simulink model "pulse_generator"  (R2021a)
(part 3 of 11)

  out_3_stop_6 : Subsystem  Tag=xps:sw_reg  AncestorBlock=xps_library/Memory/software_register  mask(swreg){io_dir=From Processor, io_delay=0, init_val=0, sample_period=1, names=reg, bitwidths=32, bin_pts=0, arith_types=0, sim_port=on, show_format=on}
      mask prompts: io_dir "I/O direction"; io_delay "I/O delay"; init_val "Initial Value"; sample_period "Sample period"; names "Bitfield names [msb...lsb]"; bitwidths "Bitfield widths"; bin_pts "Bitfield binary pts"; arith_types "Bitfield types, ufix=0, fix=1, bool=2"; sim_port "Provide sim input/output?"; show_format "Print format string?"
      mask help: A 32-bit software-accessible register. Can be divided into bitfields of varying widths and types using the fields in the block mask.
      mask init:
      | swreg_init(gcb)
      settings: AttributesFormatString=1input:uf32.0 = 32 bits
      mask TypeOptions io_dir: To Processor | From Processor
      mask Callback io_dir:
      | mask_enables = get_param(gcb, 'MaskEnables');
      | mask_names = get_param(gcb, 'MaskNames');
      | if strcmp(get_param(gcb, 'io_dir'), 'To Processor'),
      |     mask_enables{ismember(mask_names, 'sample_period')} = 'off';
      | else
      |     mask_enables{ismember(mask_names, 'sample_period')} = 'on';
      | end
      | set_param(gcb, 'MaskEnables', mask_enables);
      mask DialogControl ParameterTabVar0 Prompt: Setup
  out_3_stop_7 : Subsystem  Tag=xps:sw_reg  AncestorBlock=xps_library/Memory/software_register  mask(swreg){io_dir=From Processor, io_delay=0, init_val=0, sample_period=1, names=reg, bitwidths=32, bin_pts=0, arith_types=0, sim_port=on, show_format=on}
      mask prompts: io_dir "I/O direction"; io_delay "I/O delay"; init_val "Initial Value"; sample_period "Sample period"; names "Bitfield names [msb...lsb]"; bitwidths "Bitfield widths"; bin_pts "Bitfield binary pts"; arith_types "Bitfield types, ufix=0, fix=1, bool=2"; sim_port "Provide sim input/output?"; show_format "Print format string?"
      mask help: A 32-bit software-accessible register. Can be divided into bitfields of varying widths and types using the fields in the block mask.
      mask init:
      | swreg_init(gcb)
      settings: AttributesFormatString=1input:uf32.0 = 32 bits
      mask TypeOptions io_dir: To Processor | From Processor
      mask Callback io_dir:
      | mask_enables = get_param(gcb, 'MaskEnables');
      | mask_names = get_param(gcb, 'MaskNames');
      | if strcmp(get_param(gcb, 'io_dir'), 'To Processor'),
      |     mask_enables{ismember(mask_names, 'sample_period')} = 'off';
      | else
      |     mask_enables{ismember(mask_names, 'sample_period')} = 'on';
      | end
      | set_param(gcb, 'MaskEnables', mask_enables);
      mask DialogControl ParameterTabVar0 Prompt: Setup
  out_3_stop_8 : Subsystem  Tag=xps:sw_reg  AncestorBlock=xps_library/Memory/software_register  mask(swreg){io_dir=From Processor, io_delay=0, init_val=0, sample_period=1, names=reg, bitwidths=32, bin_pts=0, arith_types=0, sim_port=on, show_format=on}
      mask prompts: io_dir "I/O direction"; io_delay "I/O delay"; init_val "Initial Value"; sample_period "Sample period"; names "Bitfield names [msb...lsb]"; bitwidths "Bitfield widths"; bin_pts "Bitfield binary pts"; arith_types "Bitfield types, ufix=0, fix=1, bool=2"; sim_port "Provide sim input/output?"; show_format "Print format string?"
      mask help: A 32-bit software-accessible register. Can be divided into bitfields of varying widths and types using the fields in the block mask.
      mask init:
      | swreg_init(gcb)
      settings: AttributesFormatString=1input:uf32.0 = 32 bits
      mask TypeOptions io_dir: To Processor | From Processor
      mask Callback io_dir:
      | mask_enables = get_param(gcb, 'MaskEnables');
      | mask_names = get_param(gcb, 'MaskNames');
      | if strcmp(get_param(gcb, 'io_dir'), 'To Processor'),
      |     mask_enables{ismember(mask_names, 'sample_period')} = 'off';
      | else
      |     mask_enables{ismember(mask_names, 'sample_period')} = 'on';
      | end
      | set_param(gcb, 'MaskEnables', mask_enables);
      mask DialogControl ParameterTabVar0 Prompt: Setup
  out_3_stop_9 : Subsystem  Tag=xps:sw_reg  AncestorBlock=xps_library/Memory/software_register  mask(swreg){io_dir=From Processor, io_delay=0, init_val=0, sample_period=1, names=reg, bitwidths=32, bin_pts=0, arith_types=0, sim_port=on, show_format=on}
      mask prompts: io_dir "I/O direction"; io_delay "I/O delay"; init_val "Initial Value"; sample_period "Sample period"; names "Bitfield names [msb...lsb]"; bitwidths "Bitfield widths"; bin_pts "Bitfield binary pts"; arith_types "Bitfield types, ufix=0, fix=1, bool=2"; sim_port "Provide sim input/output?"; show_format "Print format string?"
      mask help: A 32-bit software-accessible register. Can be divided into bitfields of varying widths and types using the fields in the block mask.
      mask init:
      | swreg_init(gcb)
      settings: AttributesFormatString=1input:uf32.0 = 32 bits
      mask TypeOptions io_dir: To Processor | From Processor
      mask Callback io_dir:
      | mask_enables = get_param(gcb, 'MaskEnables');
      | mask_names = get_param(gcb, 'MaskNames');
      | if strcmp(get_param(gcb, 'io_dir'), 'To Processor'),
      |     mask_enables{ismember(mask_names, 'sample_period')} = 'off';
      | else
      |     mask_enables{ismember(mask_names, 'sample_period')} = 'on';
      | end
      | set_param(gcb, 'MaskEnables', mask_enables);
      mask DialogControl ParameterTabVar0 Prompt: Setup
  period : Subsystem  Tag=xps:sw_reg  AncestorBlock=xps_library/Memory/software_register  mask(swreg){io_dir=From Processor, io_delay=0, init_val=0, sample_period=1, names=reg, bitwidths=32, bin_pts=0, arith_types=0, sim_port=on, show_format=on}
      mask prompts: io_dir "I/O direction"; io_delay "I/O delay"; init_val "Initial Value"; sample_period "Sample period"; names "Bitfield names [msb...lsb]"; bitwidths "Bitfield widths"; bin_pts "Bitfield binary pts"; arith_types "Bitfield types, ufix=0, fix=1, bool=2"; sim_port "Provide sim input/output?"; show_format "Print format string?"
      mask help: A 32-bit software-accessible register. Can be divided into bitfields of varying widths and types using the fields in the block mask.
      mask init:
      | swreg_init(gcb)
      settings: AttributesFormatString=1input:uf32.0 = 32 bits
      mask TypeOptions io_dir: To Processor | From Processor
      mask Callback io_dir:
      | mask_enables = get_param(gcb, 'MaskEnables');
      | mask_names = get_param(gcb, 'MaskNames');
      | if strcmp(get_param(gcb, 'io_dir'), 'To Processor'),
      |     mask_enables{ismember(mask_names, 'sample_period')} = 'off';
      | else
      |     mask_enables{ismember(mask_names, 'sample_period')} = 'on';
      | end
      | set_param(gcb, 'MaskEnables', mask_enables);
      mask DialogControl ParameterTabVar0 Prompt: Setup
  pulse_logic_1 : Subsystem  ReferencedSubsystem=pulse_logic
  pulse_logic_2 : Subsystem  ReferencedSubsystem=pulse_logic
  pulse_logic_3 : Subsystem  ReferencedSubsystem=pulse_logic
  red_pitaya_dac : xps_library/DACs/red_pitaya_dac  Tag=xps:red_pitaya_dac  Commented=on  bits=10
      settings: SourceProductName=CASPER XPS Blockset
  reset : Subsystem  Tag=xps:sw_reg  AncestorBlock=xps_library/Memory/software_register  mask(swreg){io_dir=From Processor, io_delay=0, init_val=0, sample_period=1, names=reg, bitwidths=1, bin_pts=0, arith_types=2, sim_port=on, show_format=on}
      mask prompts: io_dir "I/O direction"; io_delay "I/O delay"; init_val "Initial Value"; sample_period "Sample period"; names "Bitfield names [msb...lsb]"; bitwidths "Bitfield widths"; bin_pts "Bitfield binary pts"; arith_types "Bitfield types, ufix=0, fix=1, bool=2"; sim_port "Provide sim input/output?"; show_format "Print format string?"
      mask help: A 32-bit software-accessible register. Can be divided into bitfields of varying widths and types using the fields in the block mask.
      mask init:
      | swreg_init(gcb)
      settings: AttributesFormatString=1input:b = 1 bits
      mask TypeOptions io_dir: To Processor | From Processor
      mask Callback io_dir:
      | mask_enables = get_param(gcb, 'MaskEnables');
      | mask_names = get_param(gcb, 'MaskNames');
      | if strcmp(get_param(gcb, 'io_dir'), 'To Processor'),
      |     mask_enables{ismember(mask_names, 'sample_period')} = 'off';
      | else
      |     mask_enables{ismember(mask_names, 'sample_period')} = 'on';
      | end
      | set_param(gcb, 'MaskEnables', mask_enables);
      mask DialogControl ParameterTabVar0 Prompt: Setup
  sum_a_b : Subsystem  Tag=xps:sw_reg  AncestorBlock=xps_library/Memory/software_register  mask(swreg){io_dir=To Processor, io_delay=0, init_val=0, sample_period=1, names=reg, bitwidths=32, bin_pts=0, arith_types=0, sim_port=on, show_format=off}
      mask prompts: io_dir "I/O direction"; io_delay "I/O delay"; init_val "Initial Value"; sample_period "Sample period"; names "Bitfield names [msb...lsb]"; bitwidths "Bitfield widths"; bin_pts "Bitfield binary pts"; arith_types "Bitfield types, ufix=0, fix=1, bool=2"; sim_port "Provide sim input/output?"; show_format "Print format string?"
      mask help: A 32-bit software-accessible register. Can be divided into bitfields of varying widths and types using the fields in the block mask.
      mask init:
      | swreg_init(gcb)
      settings: AttributesFormatString=1output
      mask TypeOptions io_dir: To Processor | From Processor
      mask Callback io_dir:
      | mask_enables = get_param(gcb, 'MaskEnables');
      | mask_names = get_param(gcb, 'MaskNames');
      | if strcmp(get_param(gcb, 'io_dir'), 'To Processor'),
      |     mask_enables{ismember(mask_names, 'sample_period')} = 'off';
      | else
      |     mask_enables{ismember(mask_names, 'sample_period')} = 'on';
      | end
      | set_param(gcb, 'MaskEnables', mask_enables);
      mask DialogControl ParameterTabVar0 Prompt: Setup
  tick_counter : Subsystem  Tag=xps:sw_reg  AncestorBlock=xps_library/Memory/software_register  mask(swreg){io_dir=To Processor, io_delay=0, init_val=0, sample_period=1, names=reg, bitwidths=32, bin_pts=0, arith_types=0, sim_port=on, show_format=off}
      mask prompts: io_dir "I/O direction"; io_delay "I/O delay"; init_val "Initial Value"; sample_period "Sample period"; names "Bitfield names [msb...lsb]"; bitwidths "Bitfield widths"; bin_pts "Bitfield binary pts"; arith_types "Bitfield types, ufix=0, fix=1, bool=2"; sim_port "Provide sim input/output?"; show_format "Print format string?"
      mask help: A 32-bit software-accessible register. Can be divided into bitfields of varying widths and types using the fields in the block mask.
      mask init:
      | swreg_init(gcb)
      settings: AttributesFormatString=1output
      mask TypeOptions io_dir: To Processor | From Processor
      mask Callback io_dir:
      | mask_enables = get_param(gcb, 'MaskEnables');
      | mask_names = get_param(gcb, 'MaskNames');
      | if strcmp(get_param(gcb, 'io_dir'), 'To Processor'),
      |     mask_enables{ismember(mask_names, 'sample_period')} = 'off';
      | else
      |     mask_enables{ismember(mask_names, 'sample_period')} = 'on';
      | end
      | set_param(gcb, 'MaskEnables', mask_enables);
      mask DialogControl ParameterTabVar0 Prompt: Setup
  wires:
  AddSub/1 -> sum_a_b/1(out_reg)
  a_sim/1 -> a/1(sim_1)
  sum_a_b/1(sim_out_reg) -> Scope1/1
  b/1(in_reg) -> AddSub/2
  b_sim/1 -> b/1(sim_1)
  a/1(in_reg) -> AddSub/1
  Constant/1 -> out_1_stop_1/1(sim_1)
  Constant1/1 -> out_1_start_1/1(sim_1)
  Delay/1 -> Scope2/2
  Counter/1 -> tick_counter/1(out_reg), [counter]
  [counter] -> Delay/1
  reset/1(in_reg) -> edge_detect/1
  Constant3/1 -> out_1_start_2/1(sim_1)
  Constant2/1 -> out_1_stop_2/1(sim_1)
  Constant6/1 -> out_1_stop_4/1(sim_1)
  Constant7/1 -> out_1_start_4/1(sim_1)
  Constant5/1 -> out_1_start_3/1(sim_1)
  Constant4/1 -> out_1_stop_3/1(sim_1)
  Constant12/1 -> out_1_stop_7/1(sim_1)
  Constant13/1 -> out_1_start_7/1(sim_1)
  Constant10/1 -> out_1_stop_6/1(sim_1)
  Constant11/1 -> out_1_start_6/1(sim_1)
  Constant9/1 -> out_1_start_5/1(sim_1)
  Constant8/1 -> out_1_stop_5/1(sim_1)
  [counter] -> pulse_logic_1/1
  pulse_logic_1/1 -> Inverter/1, led1/1
  pulse_logic_2/1 -> led2/1, Inverter1/1
  [counter] -> pulse_logic_2/1
  Constant30/1 -> out_2_stop_5/1(sim_1)
  Constant31/1 -> out_2_start_5/1(sim_1)
  Constant19/1 -> out_2_start_6/1(sim_1)
  Constant18/1 -> out_2_stop_6/1(sim_1)
  Constant21/1 -> out_2_start_7/1(sim_1)
  Constant20/1 -> out_2_stop_7/1(sim_1)
  Constant26/1 -> out_2_stop_3/1(sim_1)
  Constant27/1 -> out_2_start_3/1(sim_1)
  Constant29/1 -> out_2_start_4/1(sim_1)
  Constant28/1 -> out_2_stop_4/1(sim_1)
  Constant24/1 -> out_2_stop_2/1(sim_1)
  Constant25/1 -> out_2_start_2/1(sim_1)
  Constant17/1 -> out_2_start_1/1(sim_1)
  Constant16/1 -> out_2_stop_1/1(sim_1)
  Constant32/1 -> out_3_stop_1/1(sim_1)
  Constant33/1 -> out_3_start_1/1(sim_1)
  Constant41/1 -> out_3_start_2/1(sim_1)
  Constant40/1 -> out_3_stop_2/1(sim_1)
  Constant44/1 -> out_3_stop_4/1(sim_1)
  Constant45/1 -> out_3_start_4/1(sim_1)
  Constant43/1 -> out_3_start_3/1(sim_1)
  Constant42/1 -> out_3_stop_3/1(sim_1)
  Constant36/1 -> out_3_stop_7/1(sim_1)
  Constant37/1 -> out_3_start_7/1(sim_1)
  Constant34/1 -> out_3_stop_6/1(sim_1)
  Constant35/1 -> out_3_start_6/1(sim_1)
  Constant47/1 -> out_3_start_5/1(sim_1)
  Constant46/1 -> out_3_stop_5/1(sim_1)
  [counter] -> pulse_logic_3/1
  edge_detect/1 -> [rst]
  Constant48/1 -> period/1(sim_1)
  period/1(in_reg) -> Relational/2
  Relational/1 -> edge_detect1/1
  Logical/1 -> Counter/1
  [period_rst] -> Logical/2
  [rst] -> Logical/1
  AddSub1/1 -> Relational/1
  Constant49/1 -> AddSub1/2
  [counter] -> AddSub1/1
  Step/1 -> reset/1(sim_1)
  edge_detect1/1 -> [period_rst]
  Constant51/1 -> red_pitaya_dac/2
  From6/1 -> red_pitaya_dac/1
  pulse_logic_3/1 -> Inverter2/1, Reinterpret/1, led3/1
  Reinterpret/1 -> Shift1/1
  Shift1/1 -> red_pitaya_dac/4, red_pitaya_dac/3
  Constant52/1 -> counter_en/1(sim_1)
  AddSub2/1 -> Register/1
  Register/1 -> cycle_counter/1(out_reg), Relational1/2, AddSub2/1
  [period_rst] -> Reinterpret1/1
  [rst] -> Register/2
  out_1_start_1/1(in_reg) -> pulse_logic_1/4
  Constant15/1 -> out_1_start_0/1(sim_1)
  Constant14/1 -> out_1_stop_0/1(sim_1)
  out_1_start_0/1(in_reg) -> pulse_logic_1/2
  out_1_stop_0/1(in_reg) -> pulse_logic_1/3
  out_1_stop_1/1(in_reg) -> pulse_logic_1/5
  out_1_start_2/1(in_reg) -> pulse_logic_1/6
  out_1_start_3/1(in_reg) -> pulse_logic_1/8
  out_1_stop_2/1(in_reg) -> pulse_logic_1/7
  out_1_stop_3/1(in_reg) -> pulse_logic_1/9
  out_1_start_4/1(in_reg) -> pulse_logic_1/10
  out_1_stop_4/1(in_reg) -> pulse_logic_1/11
  out_1_start_5/1(in_reg) -> pulse_logic_1/12
  out_1_stop_5/1(in_reg) -> pulse_logic_1/13
  out_1_start_6/1(in_reg) -> pulse_logic_1/14
  out_1_stop_6/1(in_reg) -> pulse_logic_1/15
  out_1_start_7/1(in_reg) -> pulse_logic_1/16
  out_1_stop_7/1(in_reg) -> pulse_logic_1/17
  out_2_start_1/1(in_reg) -> pulse_logic_2/4
  Constant22/1 -> out_2_stop_0/1(sim_1)
  Constant23/1 -> out_2_start_0/1(sim_1)
  out_2_start_0/1(in_reg) -> pulse_logic_2/2
  out_2_stop_0/1(in_reg) -> pulse_logic_2/3
  out_2_stop_1/1(in_reg) -> pulse_logic_2/5
  out_2_start_2/1(in_reg) -> pulse_logic_2/6
  out_2_stop_2/1(in_reg) -> pulse_logic_2/7
  out_2_start_3/1(in_reg) -> pulse_logic_2/8
  out_2_stop_3/1(in_reg) -> pulse_logic_2/9
  out_2_start_4/1(in_reg) -> pulse_logic_2/10
  out_2_stop_4/1(in_reg) -> pulse_logic_2/11
  out_2_start_5/1(in_reg) -> pulse_logic_2/12
  out_2_stop_5/1(in_reg) -> pulse_logic_2/13
  out_2_start_6/1(in_reg) -> pulse_logic_2/14
  out_2_stop_6/1(in_reg) -> pulse_logic_2/15
  out_2_start_7/1(in_reg) -> pulse_logic_2/16
  out_2_stop_7/1(in_reg) -> pulse_logic_2/17
  out_3_stop_7/1(in_reg) -> pulse_logic_3/17
  Constant39/1 -> out_3_start_0/1(sim_1)
  Constant38/1 -> out_3_stop_0/1(sim_1)
  out_3_start_0/1(in_reg) -> pulse_logic_3/2
  out_3_stop_0/1(in_reg) -> pulse_logic_3/3
  out_3_stop_1/1(in_reg) -> pulse_logic_3/5
  out_3_start_2/1(in_reg) -> pulse_logic_3/6
  out_3_stop_2/1(in_reg) -> pulse_logic_3/7
  out_3_start_3/1(in_reg) -> pulse_logic_3/8
  out_3_start_1/1(in_reg) -> pulse_logic_3/4
  out_3_stop_3/1(in_reg) -> pulse_logic_3/9
  out_3_start_4/1(in_reg) -> pulse_logic_3/10
  out_3_stop_4/1(in_reg) -> pulse_logic_3/11
  out_3_start_5/1(in_reg) -> pulse_logic_3/12
  out_3_stop_5/1(in_reg) -> pulse_logic_3/13
  out_3_start_6/1(in_reg) -> pulse_logic_3/14
  out_3_stop_6/1(in_reg) -> pulse_logic_3/15
  out_3_start_7/1(in_reg) -> pulse_logic_3/16
  Reinterpret1/1 -> AddSub2/2
  tick_counter/1(sim_out_reg) -> Scope3/2
  cycle_counter/1(sim_out_reg) -> Scope3/1
  Inverter/1 -> out1/1
  Inverter1/1 -> out2/1
  Inverter2/1 -> out3/1
  out_1_stop_15/1(in_reg) -> pulse_logic_1/33
  out_1_start_15/1(in_reg) -> pulse_logic_1/32
  out_1_stop_14/1(in_reg) -> pulse_logic_1/31
  out_1_start_14/1(in_reg) -> pulse_logic_1/30
  out_1_stop_13/1(in_reg) -> pulse_logic_1/29
  out_1_start_13/1(in_reg) -> pulse_logic_1/28
  out_1_stop_12/1(in_reg) -> pulse_logic_1/27
  out_1_start_12/1(in_reg) -> pulse_logic_1/26
  out_1_stop_11/1(in_reg) -> pulse_logic_1/25
  out_1_stop_10/1(in_reg) -> pulse_logic_1/23
  out_1_start_11/1(in_reg) -> pulse_logic_1/24
  out_1_start_10/1(in_reg) -> pulse_logic_1/22
  out_1_stop_9/1(in_reg) -> pulse_logic_1/21
  out_1_stop_8/1(in_reg) -> pulse_logic_1/19
  out_1_start_8/1(in_reg) -> pulse_logic_1/18
  Constant59/1 -> out_1_stop_8/1(sim_1)
  Constant60/1 -> out_1_start_8/1(sim_1)
  out_1_start_9/1(in_reg) -> pulse_logic_1/20
  Constant67/1 -> out_1_stop_13/1(sim_1)
  Constant68/1 -> out_1_start_13/1(sim_1)
  Constant56/1 -> out_1_start_14/1(sim_1)
  Constant55/1 -> out_1_stop_14/1(sim_1)
  Constant58/1 -> out_1_start_15/1(sim_1)
  Constant57/1 -> out_1_stop_15/1(sim_1)
  Constant63/1 -> out_1_stop_11/1(sim_1)
  Constant64/1 -> out_1_start_11/1(sim_1)
  Constant66/1 -> out_1_start_12/1(sim_1)
  Constant65/1 -> out_1_stop_12/1(sim_1)
  Constant61/1 -> out_1_stop_10/1(sim_1)
  Constant62/1 -> out_1_start_10/1(sim_1)
  Constant54/1 -> out_1_start_9/1(sim_1)
  Constant53/1 -> out_1_stop_9/1(sim_1)
  out_1_stop_17/1(in_reg) -> pulse_logic_1/37
  out_1_stop_16/1(in_reg) -> pulse_logic_1/35
  out_1_start_16/1(in_reg) -> pulse_logic_1/34
  Constant75/1 -> out_1_stop_16/1(sim_1)
  Constant76/1 -> out_1_start_16/1(sim_1)
  out_1_start_17/1(in_reg) -> pulse_logic_1/36
  Constant70/1 -> out_1_start_17/1(sim_1)
  Constant69/1 -> out_1_stop_17/1(sim_1)
  Constant77/1 -> out_1_stop_21/1(sim_1)
  Constant78/1 -> out_1_start_21/1(sim_1)
  out_1_start_21/1(in_reg) -> pulse_logic_1/44
  Constant80/1 -> out_1_start_20/1(sim_1)
  Constant79/1 -> out_1_stop_20/1(sim_1)
  out_1_start_20/1(in_reg) -> pulse_logic_1/42
  out_1_stop_20/1(in_reg) -> pulse_logic_1/43
  out_1_stop_21/1(in_reg) -> pulse_logic_1/45
  Constant73/1 -> out_1_stop_19/1(sim_1)
  Constant74/1 -> out_1_start_19/1(sim_1)
  Constant71/1 -> out_1_stop_18/1(sim_1)
  Constant72/1 -> out_1_start_18/1(sim_1)
  out_1_start_18/1(in_reg) -> pulse_logic_1/38
  out_1_stop_18/1(in_reg) -> pulse_logic_1/39
  out_1_start_19/1(in_reg) -> pulse_logic_1/40
  out_1_stop_19/1(in_reg) -> pulse_logic_1/41
  Constant82/1 -> out_1_start_22/1(sim_1)
  Constant81/1 -> out_1_stop_22/1(sim_1)
  Constant84/1 -> out_1_start_23/1(sim_1)
  Constant83/1 -> out_1_stop_23/1(sim_1)
  Constant87/1 -> out_1_stop_24/1(sim_1)
  Constant88/1 -> out_1_start_24/1(sim_1)
  Constant86/1 -> out_1_start_25/1(sim_1)
  Constant85/1 -> out_1_stop_25/1(sim_1)
  out_1_start_22/1(in_reg) -> pulse_logic_1/46
  out_1_stop_22/1(in_reg) -> pulse_logic_1/47
  out_1_start_23/1(in_reg) -> pulse_logic_1/48
  out_1_stop_23/1(in_reg) -> pulse_logic_1/49
  out_1_start_24/1(in_reg) -> pulse_logic_1/50
  out_1_stop_24/1(in_reg) -> pulse_logic_1/51
  out_1_start_25/1(in_reg) -> pulse_logic_1/52
  out_1_stop_25/1(in_reg) -> pulse_logic_1/53
  out_1_stop_29/1(in_reg) -> pulse_logic_1/61
  out_1_start_29/1(in_reg) -> pulse_logic_1/60
  out_1_stop_28/1(in_reg) -> pulse_logic_1/59
  out_1_start_28/1(in_reg) -> pulse_logic_1/58
  out_1_stop_27/1(in_reg) -> pulse_logic_1/57
  out_1_start_27/1(in_reg) -> pulse_logic_1/56
  out_1_stop_26/1(in_reg) -> pulse_logic_1/55
  out_1_start_26/1(in_reg) -> pulse_logic_1/54
  Constant93/1 -> out_1_stop_29/1(sim_1)
  Constant94/1 -> out_1_start_29/1(sim_1)
  Constant96/1 -> out_1_start_28/1(sim_1)
  Constant95/1 -> out_1_stop_28/1(sim_1)
  Constant91/1 -> out_1_stop_27/1(sim_1)
  Constant92/1 -> out_1_start_27/1(sim_1)
  Constant89/1 -> out_1_stop_26/1(sim_1)
  Constant90/1 -> out_1_start_26/1(sim_1)
  Constant99/1 -> out_1_stop_30/1(sim_1)
  Constant100/1 -> out_1_start_30/1(sim_1)
  Constant98/1 -> out_1_start_31/1(sim_1)
  Constant97/1 -> out_1_stop_31/1(sim_1)
  out_1_start_30/1(in_reg) -> pulse_logic_1/62
  out_1_stop_30/1(in_reg) -> pulse_logic_1/63
  out_1_start_31/1(in_reg) -> pulse_logic_1/64
  out_1_stop_31/1(in_reg) -> pulse_logic_1/65
  out_2_stop_15/1(in_reg) -> pulse_logic_2/33
  out_2_start_15/1(in_reg) -> pulse_logic_2/32
  out_2_stop_14/1(in_reg) -> pulse_logic_2/31
  out_2_start_14/1(in_reg) -> pulse_logic_2/30
  out_2_stop_13/1(in_reg) -> pulse_logic_2/29
  out_2_start_13/1(in_reg) -> pulse_logic_2/28
  out_2_stop_12/1(in_reg) -> pulse_logic_2/27
  out_2_start_12/1(in_reg) -> pulse_logic_2/26
  out_2_stop_11/1(in_reg) -> pulse_logic_2/25
  out_2_start_11/1(in_reg) -> pulse_logic_2/24
  out_2_stop_10/1(in_reg) -> pulse_logic_2/23
  out_2_start_10/1(in_reg) -> pulse_logic_2/22
  out_2_stop_9/1(in_reg) -> pulse_logic_2/21
  out_2_stop_8/1(in_reg) -> pulse_logic_2/19
  out_2_start_8/1(in_reg) -> pulse_logic_2/18
  Constant108/1 -> out_2_start_8/1(sim_1)
  Constant107/1 -> out_2_stop_8/1(sim_1)
  out_2_start_9/1(in_reg) -> pulse_logic_2/20
  Constant101/1 -> out_2_stop_9/1(sim_1)
  Constant102/1 -> out_2_start_9/1(sim_1)
  Constant110/1 -> out_2_start_10/1(sim_1)
  Constant109/1 -> out_2_stop_10/1(sim_1)
  Constant113/1 -> out_2_stop_12/1(sim_1)
  Constant114/1 -> out_2_start_12/1(sim_1)
  Constant112/1 -> out_2_start_11/1(sim_1)
  Constant111/1 -> out_2_stop_11/1(sim_1)
  Constant105/1 -> out_2_stop_15/1(sim_1)
  Constant106/1 -> out_2_start_15/1(sim_1)
  Constant103/1 -> out_2_stop_14/1(sim_1)
  Constant104/1 -> out_2_start_14/1(sim_1)
  Constant116/1 -> out_2_start_13/1(sim_1)
  Constant115/1 -> out_2_stop_13/1(sim_1)
  Constant123/1 -> out_2_stop_17/1(sim_1)
  Constant124/1 -> out_2_start_17/1(sim_1)
  Constant118/1 -> out_2_start_18/1(sim_1)
  Constant117/1 -> out_2_stop_18/1(sim_1)
  Constant120/1 -> out_2_start_19/1(sim_1)
  Constant119/1 -> out_2_stop_19/1(sim_1)
  Constant122/1 -> out_2_start_16/1(sim_1)
  Constant121/1 -> out_2_stop_16/1(sim_1)
  out_2_start_16/1(in_reg) -> pulse_logic_2/34
  out_2_stop_16/1(in_reg) -> pulse_logic_2/35
  out_2_start_17/1(in_reg) -> pulse_logic_2/36
  out_2_stop_17/1(in_reg) -> pulse_logic_2/37
  out_2_start_18/1(in_reg) -> pulse_logic_2/38
  out_2_stop_18/1(in_reg) -> pulse_logic_2/39
  out_2_start_19/1(in_reg) -> pulse_logic_2/40
  out_2_stop_19/1(in_reg) -> pulse_logic_2/41
  out_2_stop_23/1(in_reg) -> pulse_logic_2/49
  out_2_start_23/1(in_reg) -> pulse_logic_2/48
  out_2_stop_22/1(in_reg) -> pulse_logic_2/47
  out_2_start_22/1(in_reg) -> pulse_logic_2/46
  out_2_stop_21/1(in_reg) -> pulse_logic_2/45
  out_2_start_21/1(in_reg) -> pulse_logic_2/44
  out_2_stop_20/1(in_reg) -> pulse_logic_2/43
  out_2_start_20/1(in_reg) -> pulse_logic_2/42
  Constant129/1 -> out_2_stop_20/1(sim_1)
  Constant130/1 -> out_2_start_20/1(sim_1)
  Constant127/1 -> out_2_stop_23/1(sim_1)
  Constant128/1 -> out_2_start_23/1(sim_1)
  Constant125/1 -> out_2_stop_22/1(sim_1)
  Constant126/1 -> out_2_start_22/1(sim_1)
  Constant132/1 -> out_2_start_21/1(sim_1)
  Constant131/1 -> out_2_stop_21/1(sim_1)
  Constant139/1 -> out_2_stop_25/1(sim_1)
  Constant140/1 -> out_2_start_25/1(sim_1)
  Constant134/1 -> out_2_start_26/1(sim_1)
  Constant133/1 -> out_2_stop_26/1(sim_1)
  Constant136/1 -> out_2_start_27/1(sim_1)
  Constant135/1 -> out_2_stop_27/1(sim_1)
  Constant138/1 -> out_2_start_24/1(sim_1)
  Constant137/1 -> out_2_stop_24/1(sim_1)
  out_2_start_24/1(in_reg) -> pulse_logic_2/50
  out_2_stop_24/1(in_reg) -> pulse_logic_2/51
  out_2_start_25/1(in_reg) -> pulse_logic_2/52
  out_2_stop_25/1(in_reg) -> pulse_logic_2/53
  out_2_start_26/1(in_reg) -> pulse_logic_2/54
  out_2_stop_26/1(in_reg) -> pulse_logic_2/55
  out_2_start_27/1(in_reg) -> pulse_logic_2/56
  out_2_stop_27/1(in_reg) -> pulse_logic_2/57
  out_2_stop_31/1(in_reg) -> pulse_logic_2/65
  out_2_start_31/1(in_reg) -> pulse_logic_2/64
  out_2_stop_30/1(in_reg) -> pulse_logic_2/63
  out_2_start_30/1(in_reg) -> pulse_logic_2/62
  out_2_stop_29/1(in_reg) -> pulse_logic_2/61
  out_2_start_29/1(in_reg) -> pulse_logic_2/60
  out_2_stop_28/1(in_reg) -> pulse_logic_2/59
  out_2_start_28/1(in_reg) -> pulse_logic_2/58
  Constant145/1 -> out_2_stop_28/1(sim_1)
  Constant146/1 -> out_2_start_28/1(sim_1)
  Constant143/1 -> out_2_stop_31/1(sim_1)
  Constant144/1 -> out_2_start_31/1(sim_1)
  Constant141/1 -> out_2_stop_30/1(sim_1)
  Constant142/1 -> out_2_start_30/1(sim_1)
  Constant148/1 -> out_2_start_29/1(sim_1)
  Constant147/1 -> out_2_stop_29/1(sim_1)
  out_3_start_15/1(in_reg) -> pulse_logic_3/32
  out_3_stop_14/1(in_reg) -> pulse_logic_3/31
  out_3_start_14/1(in_reg) -> pulse_logic_3/30
  out_3_stop_13/1(in_reg) -> pulse_logic_3/29
  out_3_start_13/1(in_reg) -> pulse_logic_3/28
  out_3_stop_12/1(in_reg) -> pulse_logic_3/27
  out_3_start_12/1(in_reg) -> pulse_logic_3/26
  out_3_stop_11/1(in_reg) -> pulse_logic_3/25
  out_3_start_9/1(in_reg) -> pulse_logic_3/20
  out_3_start_11/1(in_reg) -> pulse_logic_3/24
  out_3_stop_10/1(in_reg) -> pulse_logic_3/23
  out_3_start_10/1(in_reg) -> pulse_logic_3/22
  out_3_stop_9/1(in_reg) -> pulse_logic_3/21
  out_3_stop_8/1(in_reg) -> pulse_logic_3/19
  out_3_start_8/1(in_reg) -> pulse_logic_3/18
  Constant155/1 -> out_3_stop_8/1(sim_1)
  Constant156/1 -> out_3_start_8/1(sim_1)
  out_3_stop_15/1(in_reg) -> pulse_logic_3/33
  Constant163/1 -> out_3_stop_13/1(sim_1)
  Constant164/1 -> out_3_start_13/1(sim_1)
  Constant152/1 -> out_3_start_14/1(sim_1)
  Constant151/1 -> out_3_stop_14/1(sim_1)
  Constant154/1 -> out_3_start_15/1(sim_1)
  Constant153/1 -> out_3_stop_15/1(sim_1)
  Constant159/1 -> out_3_stop_11/1(sim_1)
  Constant160/1 -> out_3_start_11/1(sim_1)
  Constant162/1 -> out_3_start_12/1(sim_1)
  Constant161/1 -> out_3_stop_12/1(sim_1)
  Constant157/1 -> out_3_stop_10/1(sim_1)
  Constant158/1 -> out_3_start_10/1(sim_1)
  Constant150/1 -> out_3_start_9/1(sim_1)
  Constant149/1 -> out_3_stop_9/1(sim_1)
  Constant169/1 -> out_3_stop_16/1(sim_1)
  Constant170/1 -> out_3_start_16/1(sim_1)
  Constant167/1 -> out_3_stop_19/1(sim_1)
  Constant168/1 -> out_3_start_19/1(sim_1)
  Constant165/1 -> out_3_stop_18/1(sim_1)
  Constant166/1 -> out_3_start_18/1(sim_1)
  Constant172/1 -> out_3_start_17/1(sim_1)
  Constant171/1 -> out_3_stop_17/1(sim_1)
  out_3_stop_19/1(in_reg) -> pulse_logic_3/41
  out_3_start_16/1(in_reg) -> pulse_logic_3/34
  out_3_stop_16/1(in_reg) -> pulse_logic_3/35
  out_3_start_17/1(in_reg) -> pulse_logic_3/36
  out_3_stop_17/1(in_reg) -> pulse_logic_3/37
  out_3_start_18/1(in_reg) -> pulse_logic_3/38
  out_3_stop_18/1(in_reg) -> pulse_logic_3/39
  out_3_start_19/1(in_reg) -> pulse_logic_3/40
  out_3_start_23/1(in_reg) -> pulse_logic_3/48
  out_3_stop_22/1(in_reg) -> pulse_logic_3/47
  out_3_start_22/1(in_reg) -> pulse_logic_3/46
  out_3_stop_21/1(in_reg) -> pulse_logic_3/45
  out_3_start_21/1(in_reg) -> pulse_logic_3/44
  out_3_stop_20/1(in_reg) -> pulse_logic_3/43
  out_3_start_20/1(in_reg) -> pulse_logic_3/42
  out_3_stop_23/1(in_reg) -> pulse_logic_3/49
  Constant179/1 -> out_3_stop_21/1(sim_1)
  Constant180/1 -> out_3_start_21/1(sim_1)
  Constant174/1 -> out_3_start_22/1(sim_1)
  Constant173/1 -> out_3_stop_22/1(sim_1)
  Constant176/1 -> out_3_start_23/1(sim_1)
  Constant175/1 -> out_3_stop_23/1(sim_1)
  Constant178/1 -> out_3_start_20/1(sim_1)
  Constant177/1 -> out_3_stop_20/1(sim_1)
  Constant185/1 -> out_3_stop_24/1(sim_1)
  Constant186/1 -> out_3_start_24/1(sim_1)
  Constant183/1 -> out_3_stop_27/1(sim_1)
  Constant184/1 -> out_3_start_27/1(sim_1)
  Constant181/1 -> out_3_stop_26/1(sim_1)
  Constant182/1 -> out_3_start_26/1(sim_1)
  Constant188/1 -> out_3_start_25/1(sim_1)
  Constant187/1 -> out_3_stop_25/1(sim_1)
  out_3_stop_27/1(in_reg) -> pulse_logic_3/57
  out_3_start_24/1(in_reg) -> pulse_logic_3/50
  out_3_stop_24/1(in_reg) -> pulse_logic_3/51
  out_3_start_25/1(in_reg) -> pulse_logic_3/52
  out_3_stop_25/1(in_reg) -> pulse_logic_3/53
  out_3_start_26/1(in_reg) -> pulse_logic_3/54
  out_3_stop_26/1(in_reg) -> pulse_logic_3/55
  out_3_start_27/1(in_reg) -> pulse_logic_3/56
  out_3_start_31/1(in_reg) -> pulse_logic_3/64
  out_3_stop_30/1(in_reg) -> pulse_logic_3/63
  out_3_start_30/1(in_reg) -> pulse_logic_3/62
  out_3_stop_29/1(in_reg) -> pulse_logic_3/61
  out_3_start_29/1(in_reg) -> pulse_logic_3/60
  out_3_stop_28/1(in_reg) -> pulse_logic_3/59
  out_3_start_28/1(in_reg) -> pulse_logic_3/58
  out_3_stop_31/1(in_reg) -> pulse_logic_3/65
  Constant195/1 -> out_3_stop_29/1(sim_1)
  Constant196/1 -> out_3_start_29/1(sim_1)
  Constant190/1 -> out_3_start_30/1(sim_1)
  Constant189/1 -> out_3_stop_30/1(sim_1)
  Constant192/1 -> out_3_start_31/1(sim_1)
  Constant191/1 -> out_3_stop_31/1(sim_1)
  Constant194/1 -> out_3_start_28/1(sim_1)
  Constant193/1 -> out_3_stop_28/1(sim_1)
  counter_en/1(in_reg) -> Logical1/1
  Logical1/1 -> is_running/1(out_reg), Counter/2
  max_cycles/1(in_reg) -> Relational1/1
  Relational1/1 -> Logical2/2
  [cycle_limiter] -> Logical1/2
  Constant197/1 -> max_cycles/1(sim_1)
  out3/1 -> Scope2/1
  en_cycle_limit/1(in_reg) -> Inverter3/1
  Logical2/1 -> [cycle_limiter]
  Constant50/1 -> en_cycle_limit/1(sim_1)
  Inverter3/1 -> Logical2/1
